simulink model "Lab10"  (R2017a)
settings: Solver=VariableStepAuto  StartTime=0.0  StopTime=0.5  MaxStep=0.001000001  MinStep=0.001  RelTol=1e-5
undefined symbols (not defined in the file): ip, Js, K_d, K_y, Ka, ke, Ki, km, Ku, Kw, Mcm, T_y, T_ya, U
settings Model: Creator=User  LastModifiedBy=User

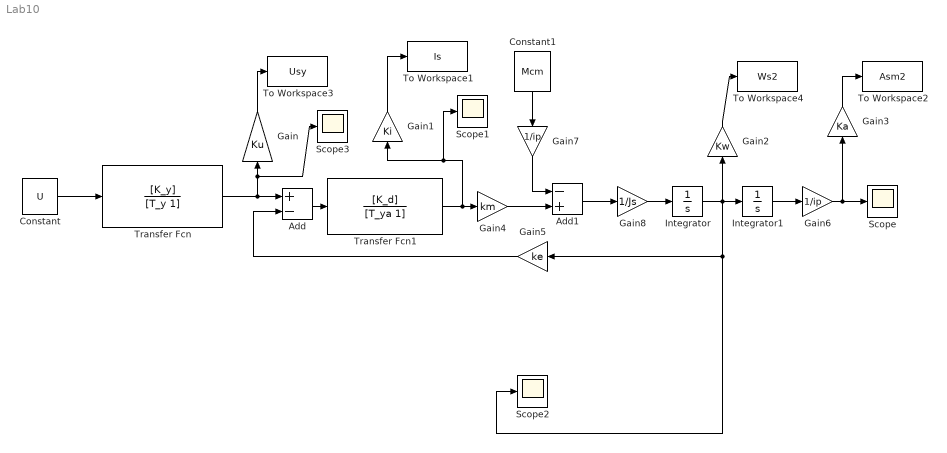
== system Lab10 ==
  Add : Sum  Inputs=+-
  Add1 : Sum  Inputs=-+
  Constant : Constant  Value=U
  Constant1 : Constant  Value=Mcm
  Gain : Gain  Gain=Ku
  Gain1 : Gain  Gain=Ki
  Gain2 : Gain  Gain=Kw
  Gain3 : Gain  Gain=Ka
  Gain4 : Gain  Gain=km
  Gain5 : Gain  Gain=ke
  Gain6 : Gain  Gain=1/ip
  Gain7 : Gain  Gain=1/ip
  Gain8 : Gain  Gain=1/Js
  Integrator : Integrator
  Integrator1 : Integrator
  Scope{,1..3} (4 alike) : Scope
  To Workspace1 : ToWorkspace  VariableName=Is  SampleTime=-1
  To Workspace2 : ToWorkspace  VariableName=Asm2  SampleTime=-1
  To Workspace3 : ToWorkspace  VariableName=Usy  SampleTime=-1
  To Workspace4 : ToWorkspace  VariableName=Ws2  SampleTime=-1
  Transfer Fcn : TransferFcn  Numerator=[K_y]  Denominator=[T_y 1]
  Transfer Fcn1 : TransferFcn  Numerator=[K_d]  Denominator=[T_ya 1]
  wires:
  Constant/1 -> Transfer Fcn/1
  Transfer Fcn/1 -> Scope3/1, Gain/1, Add/1
  Add/1 -> Transfer Fcn1/1
  Gain4/1 -> Add1/2
  Constant1/1 -> Gain7/1
  Gain7/1 -> Add1/1
  Gain/1 -> To Workspace3/1
  Transfer Fcn1/1 -> Scope1/1, Gain1/1, Gain4/1
  Gain1/1 -> To Workspace1/1
  Add1/1 -> Gain8/1
  Gain8/1 -> Integrator/1
  Integrator/1 -> Scope2/1, Gain5/1, Gain2/1, Integrator1/1
  Integrator1/1 -> Gain6/1
  Gain2/1 -> To Workspace4/1
  Gain5/1 -> Add/2
  Gain6/1 -> Scope/1, Gain3/1
  Gain3/1 -> To Workspace2/1
